simulink model "Mass_Flow"  (R2022a)
settings: Solver=VariableStepAuto  StartTime=0.0  StopTime=10.0  RelTol=1e-3
libraries: simulink x4, mbedblockslib x1
settings Model: Creator=smith  LastModifiedBy=FUGAZI

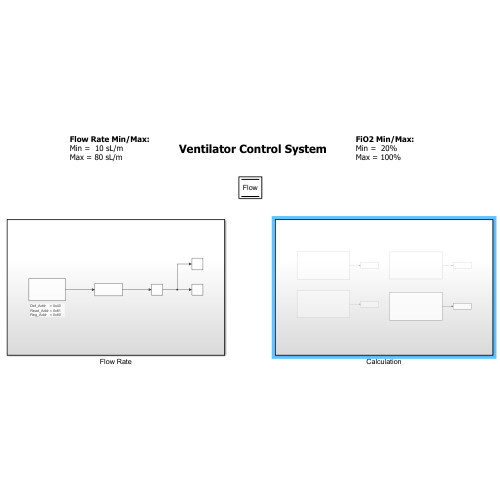
[thumbnail: Simulink's stored preview of the top-level diagram]
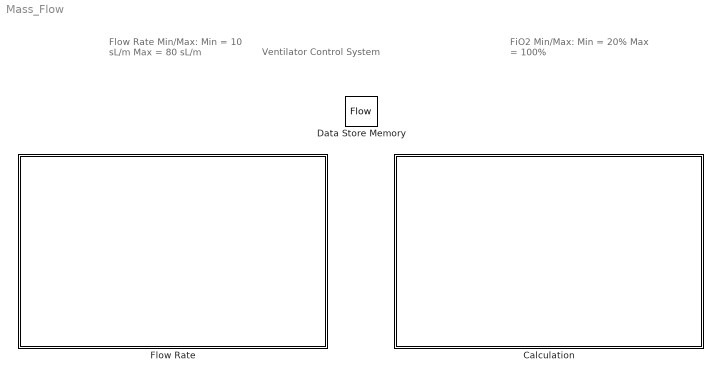
== system Mass_Flow ==
  note: Flow Rate Min/Max:
      | Min = 10 sL/m
      | Max = 80 sL/m
  note: Ventilator Control System
  note: FiO2 Min/Max:
      | Min = 20%
      | Max = 100%
  Calculation : Subsystem
  Data Store Memory : DataStoreMemory  DataStoreName=Flow  WriteAfterWriteMsg=warning  ShowAdditionalParam=off
  Flow Rate : Subsystem

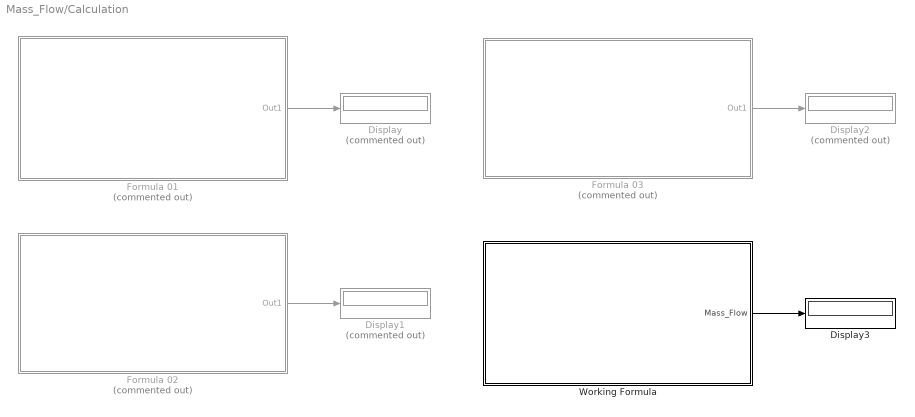
== system Mass_Flow/Calculation ==
  Display : Display  Commented=on
  Display1 : Display  Commented=on
  Display2 : Display  Commented=on
  Display3 : Display
  Formula 01 : Subsystem  Commented=on
  Formula 02 : Subsystem  Commented=on
  Formula 03 : Subsystem  Commented=on
  Working Formula : Subsystem
  wires:
  Working Formula/1(Mass_Flow) -> Display3/1
  Formula 01/1(Out1) -> Display/1
  Formula 03/1(Out1) -> Display2/1
  Formula 02/1(Out1) -> Display1/1

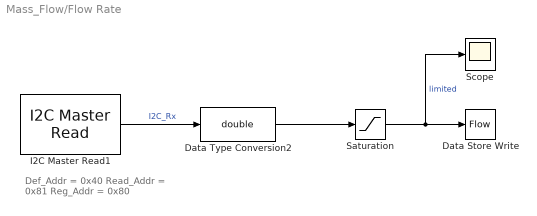
== system Mass_Flow/Flow Rate ==
  note: Def_Addr = 0x40
      | Read_Addr = 0x81
      | Reg_Addr = 0x80
  Data Store Write : DataStoreWrite  DataStoreName=Flow  IndexOptions=Index vector (dialog)  Indices=1  OutputSizes=1
  Data Type Conversion2 : DataTypeConversion  OutDataTypeStr=double  SaturateOnIntegerOverflow=off  RndMeth=Floor
  I2C Master Read1 : mbedblockslib/I2C Master Read  I2CModule=0  Mode=Master  SlaveAddress=hex2dec('0x11')  SlaveByteOrder=BigEndian  Direction=Receiver  RegisterAddressMode=off  RegisterAddress=uint8(1)  SlaveDataType=uint8  DataLength=1  NoAck=off  RepeatedStart=off  OutputStatus=off  SampleTime=0.1
      settings: SourceProductBaseCode=MICROBIT,NUCLEO,STMICRODIS
  Saturation : Saturate  UpperLimit=255  LowerLimit=-255
  Scope : Scope
  wires:
  Saturation/1 -> Data Store Write/1, Scope/1  "limited"
  I2C Master Read1/1 -> Data Type Conversion2/1  "I2C_Rx"
  Data Type Conversion2/1 -> Saturation/1

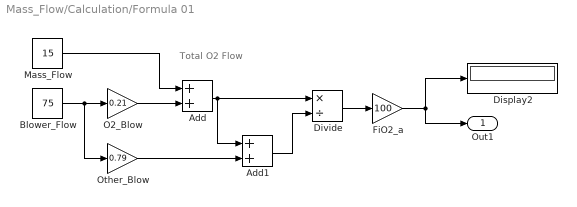
== system Mass_Flow/Calculation/Formula 01 ==
  note: Total
      | O2 Flow
  Add : Sum
  Add1 : Sum
  Blower_Flow : Constant  Value=75
  Display2 : Display
  Divide : Product  Inputs=*/
  FiO2_a : Gain  Gain=100
  Mass_Flow : Constant  Value=15
  O2_Blow : Gain  Gain=0.21
  Other_Blow : Gain  Gain=0.79
  Out1 : Outport
  wires:
  Divide/1 -> FiO2_a/1
  FiO2_a/1 -> Out1/1, Display2/1
  O2_Blow/1 -> Add/2
  Mass_Flow/1 -> Add/1
  Blower_Flow/1 -> Other_Blow/1, O2_Blow/1
  Add/1 -> Add1/1, Divide/1
  Add1/1 -> Divide/2
  Other_Blow/1 -> Add1/2

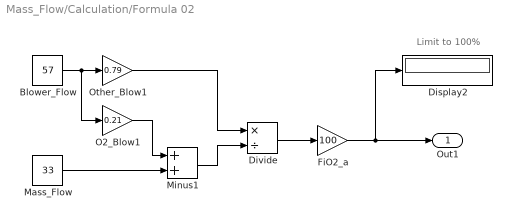
== system Mass_Flow/Calculation/Formula 02 ==
  note: Limit to 100%
  Blower_Flow : Constant  Value=57
  Display2 : Display
  Divide : Product  Inputs=*/
  FiO2_a : Gain  Gain=100
  Mass_Flow : Constant  Value=33
  Minus1 : Sum
  O2_Blow1 : Gain  Gain=0.21
  Other_Blow1 : Gain  Gain=0.79
  Out1 : Outport
  wires:
  Minus1/1 -> Divide/2
  FiO2_a/1 -> Out1/1, Display2/1
  Divide/1 -> FiO2_a/1
  Blower_Flow/1 -> O2_Blow1/1, Other_Blow1/1
  O2_Blow1/1 -> Minus1/1
  Other_Blow1/1 -> Divide/1
  Mass_Flow/1 -> Minus1/2

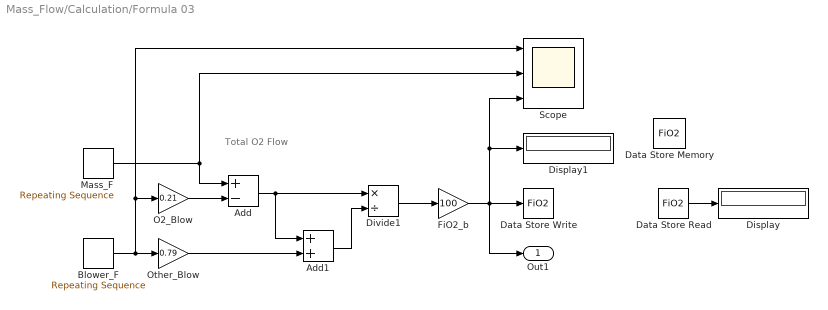
== system Mass_Flow/Calculation/Formula 03 ==
  note: Total
      | O2 Flow
  Add : Sum  Inputs=+-
  Add1 : Sum
  Blower_F : simulink/Sources/Repeating Sequence  rep_seq_t=[0 1 1.1 2 2.1 3 3.1 4 4.1]  rep_seq_y=[20 20 50 50 35 35 45 45 20]
  Data Store Memory : DataStoreMemory  DataStoreName=FiO2  WriteAfterWriteMsg=warning  ShowAdditionalParam=off
  Data Store Read : DataStoreRead  DataStoreName=FiO2  IndexOptions=Index vector (dialog)  Indices=1  OutputSizes=1
  Data Store Write : DataStoreWrite  DataStoreName=FiO2  IndexOptions=Index vector (dialog)  Indices=1  OutputSizes=1
  Display : Display
  Display1 : Display
  Divide1 : Product  Inputs=*/
  FiO2_b : Gain  Gain=100
  Mass_F : simulink/Sources/Repeating Sequence  rep_seq_t=[0 1 1.1 2 2.1 3 3.1 4 4.1]  rep_seq_y=[10 10 25 25 50 50 40 40 10]
  O2_Blow : Gain  Gain=0.21
  Other_Blow : Gain  Gain=0.79
  Scope : Scope  NumInputPorts=3
  Out1 : Outport
  wires:
  Data Store Read/1 -> Display/1
  FiO2_b/1 -> Scope/3, Display1/1, Data Store Write/1, Out1/1
  Divide1/1 -> FiO2_b/1
  Blower_F/1 -> Scope/1, O2_Blow/1, Other_Blow/1
  Mass_F/1 -> Scope/2, Add/1
  Add/1 -> Divide1/1, Add1/1
  Other_Blow/1 -> Add1/2
  O2_Blow/1 -> Add/2
  Add1/1 -> Divide1/2

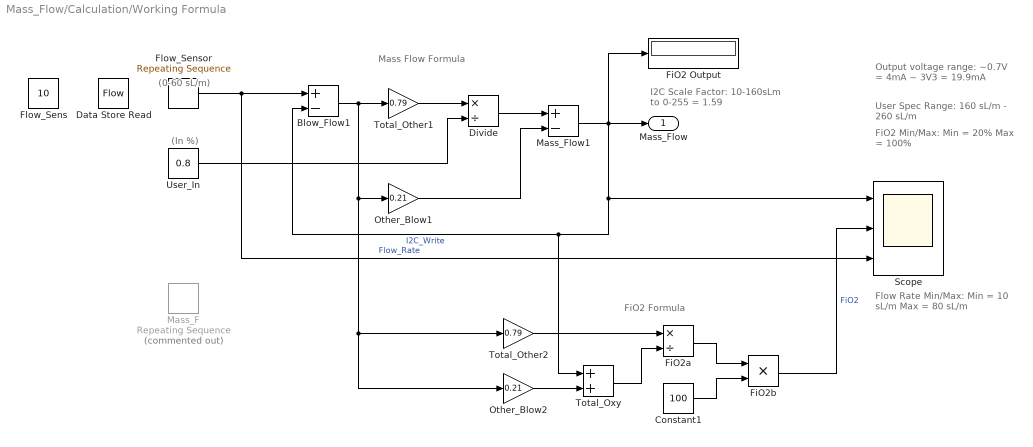
== system Mass_Flow/Calculation/Working Formula ==
  note: (In %)
  note: FiO2 Formula
  note: FiO2 Min/Max:
      | Min = 20%
      | Max = 100%
  note: Flow Rate Min/Max:
      | Min = 10 sL/m
      | Max = 80 sL/m
  note: Mass Flow Formula
  note: User Spec Range:
      | 160 sL/m - 260 sL/m
  note: Output voltage range:
      | ~0.7V = 4mA
      | ~ 3V3 = 19.9mA
  note: I2C Scale Factor:
      | 10-160sLm to 0-255 = 1.59
  note: (0-60 sL/m)
  Blow_Flow1 : Sum  Inputs=+-
  Constant1 : Constant  Value=100
  Data Store Read : DataStoreRead  DataStoreName=Flow  IndexOptions=Index vector (dialog)  Indices=1  OutputSizes=1
  Divide : Product  Inputs=*/
  FiO2 Output : Display
  FiO2a : Product  Inputs=*/
  FiO2b : Product
  Flow_Sens : Constant  Value=10
  Flow_Sensor : simulink/Sources/Repeating Sequence  rep_seq_t=[0 1 1.1 2 2.1 3 3.1 4 4.1]  rep_seq_y=[20 20 50 50 35 35 45 45 20]
  Mass_F : simulink/Sources/Repeating Sequence  Commented=on  rep_seq_t=[0 1 1.1 2 2.1 3 3.1 4 4.1]  rep_seq_y=[10 10 25 25 50 50 40 40 10]
  Mass_Flow1 : Sum  Inputs=+-
  Other_Blow1 : Gain  Gain=0.21
  Other_Blow2 : Gain  Gain=0.21
  Scope : Scope  NumInputPorts=3
  Total_Other1 : Gain  Gain=0.79
  Total_Other2 : Gain  Gain=0.79
  Total_Oxy : Sum
  User_In : Constant  Value=0.8
  Mass_Flow : Outport
  wires:
  Constant1/1 -> FiO2b/2
  User_In/1 -> Divide/2
  Total_Other1/1 -> Divide/1
  Divide/1 -> Mass_Flow1/1
  Other_Blow1/1 -> Mass_Flow1/2
  Mass_Flow1/1 -> FiO2 Output/1, Scope/1, Total_Oxy/1, Blow_Flow1/2, Mass_Flow/1  "I2C_Write"
  FiO2a/1 -> FiO2b/1
  Other_Blow2/1 -> Total_Oxy/2
  Total_Oxy/1 -> FiO2a/2
  Total_Other2/1 -> FiO2a/1
  Flow_Sensor/1 -> Scope/3, Blow_Flow1/1  "Flow_Rate"
  FiO2b/1 -> Scope/2  "FiO2"
  Blow_Flow1/1 -> Other_Blow2/1, Total_Other2/1, Other_Blow1/1, Total_Other1/1
